simulink model "ModeInputHandle"  (R2018b)
settings: Solver=FixedStepDiscrete  StartTime=0.0  StopTime=10.0  FixedStep=0.01  RelTol=1e-3
undefined symbols (not defined in the file or in its folder): c, CmprtMdHMIReqExt2Tp1, CmprtMdHMIReqExtTp1, CmprtMdHMIReqTp1, d, e, EZESwReq1, f, g, IfVeSMSeStNumConfig, j, KeSMSuButtonLongPressedThrshldTm_Val, KeSMSuFoldType_Val, KeSMSwSeatSMSSeatMdTrigGapTimer_Val, KeSMSwSeatTrigWaitTimer_Val, KeSMSwSRSActiveValidTm_Val, LckUlckActvtFunc1, LstLckFunc1, LugSelectSw1, MdReqTp1, PowerMode1, SeatOccupiedSts1, SRSMode1, StPassCmprtMdCtrl_Md10_VCUConfig_Val, StPassCmprtMdCtrl_Md11_VCUConfig_Val, StPassCmprtMdCtrl_Md12_VCUConfig_Val, StPassCmprtMdCtrl_Md13_VCUConfig_Val, StPassCmprtMdCtrl_Md1_VCUConfig_Val, StPassCmprtMdCtrl_Md27_VCUConfig_Val, StPassCmprtMdCtrl_Md28_VCUConfig_Val, StPassCmprtMdCtrl_Md29_VCUConfig_Val, StPassCmprtMdCtrl_Md2_VCUConfig_Val, StPassCmprtMdCtrl_Md30_VCUConfig_Val, StPassCmprtMdCtrl_Md31_VCUConfig_Val, StPassCmprtMdCtrl_Md32_VCUConfig_Val, StPassCmprtMdCtrl_Md3_VCUConfig_Val, StPassCmprtMdCtrl_Md53_VCUConfig_Val, StPassCmprtMdCtrl_Md56_VCUConfig_Val, StPassCmprtMdCtrl_Md57_VCUConfig_Val, StPassCmprtMdCtrl_Md58_VCUConfig_Val, StPassCmprtMdCtrl_Md61_VCUConfig_Val, StPassCmprtMdCtrl_Md62_VCUConfig_Val, StPassCmprtMdCtrl_Md8_VCUConfig_Val, StPassCmprtMdCtrl_Md9_VCUConfig_Val, StSrv_StMd10_Config_Val, StSrv_StMd11_Config_Val, StSrv_StMd12_Config_Val, StSrv_StMd13_Config_Val, StSrv_StMd1_Config_Val, StSrv_StMd27_Config_Val, StSrv_StMd28_Config_Val, StSrv_StMd29_Config_Val, StSrv_StMd2_Config_Val, StSrv_StMd30_Config_Val, StSrv_StMd31_Config_Val, StSrv_StMd32_Config_Val, StSrv_StMd3_Config_Val, StSrv_StMd8_Config_Val, StSrv_StMd9_Config_Val, VehMovState1
libraries: MSMLib x91
(part 5 of 9)

== system ModeInputHandle/ModelInputHandleRunnable_sys/Subsystem1/AcsEntry4s2RMdReq  ==
  note: // PassAcsEntry4s2RReq ---》 remote
  SwRtRclReq : Inport
  SwRtRclReqV : Inport  Port=2
  AcsEntry4s2RHMI2RRclReq : Inport  Port=3
  PassAcsEntry4s2RReq : Inport  Port=4
  PassCmprtMdHMIReqExt : Inport  Port=5
  SRSSlctSwReq : Inport  Port=6
  SRSCnfmSwReq : Inport  Port=7
  buttonLongPressedThrshhldTm : Inport  Port=8
  curMode : Inport  Port=9
  SRSActiveValidTm : Inport  Port=10
  AcsEntry4s2RAvl : Inport  Port=11
  SRSMode : Inport  Port=12
  AcsEntry4s2RMdConfig : Inport  Port=13
  AND{,1..2,4..5} (5 alike) : Logic  AllPortsSameDT=off  OutDataTypeStr=boolean
  ButtonLongPressed : Subsystem  AncestorBlock=MSMLib/ButtonLongPressed
  ButtonLongPressed2 : Subsystem  AncestorBlock=MSMLib/ButtonLongPressed
  ConfirmRequireSource : MSMLib/ConfirmRequireSource  SystemSampleTime=-1
  Constant : Constant  Value=MdReqTp1.MdReqTp_Start
  Constant1 : Constant  Value=SRSMode1.SRSSlctSwStat_EzeEntry4s2R  OutDataTypeStr=Enum:SRSMode1
  Constant2 : Constant  Value=CmprtMdHMIReqExtTp1.CmprtMdHMIReqExtTp_Mode23  OutDataTypeStr=Enum:CmprtMdHMIReqExtTp1
  Constant3 : Constant  Value=CmprtMdHMIReqExtTp1.CmprtMdHMIReqExtTp_NoAction  OutDataTypeStr=Enum:CmprtMdHMIReqExtTp1
  Constant4 : Constant  Value=true  OutDataTypeStr=boolean
  Constant5 : Constant  Value=0  OutDataTypeStr=uint8
  Constant8 : Constant  Value=9  OutDataTypeStr=uint8
  Equal : RelationalOperator  Operator===  OutDataTypeStr=boolean  RndMeth=Simplest
  Equal1 : RelationalOperator  Operator=~=  OutDataTypeStr=boolean  RndMeth=Simplest
  Equal2 : RelationalOperator  Operator===  OutDataTypeStr=boolean  RndMeth=Simplest
  Equal3 : RelationalOperator  Operator=~=  OutDataTypeStr=boolean  RndMeth=Simplest
  Equal4 : RelationalOperator  Operator===  OutDataTypeStr=boolean  RndMeth=Simplest
  Equal5 : RelationalOperator  Operator=~=  OutDataTypeStr=boolean  RndMeth=Simplest
  Ground2 : Ground
  Logical Operator : Logic  Operator=OR  Inputs=5  AllPortsSameDT=off  OutDataTypeStr=boolean
  NOT : Logic  Operator=NOT  AllPortsSameDT=off  OutDataTypeStr=boolean
  OR1 : Logic  Operator=OR  Inputs=3  AllPortsSameDT=off  OutDataTypeStr=boolean
  Relational Operator3 : RelationalOperator  Operator===  OutDataTypeStr=boolean  RndMeth=Simplest
  SRSReq : MSMLib/SRSReq  SystemSampleTime=-1
  SWIntSrc_S : MSMLib/SWIntSrc_S  SystemSampleTime=-1
  Subsystem4 : MSMLib/MergeReqAndValidity  SystemSampleTime=-1
  Switch1 : Switch  Criteria=u2 > Threshold
  Switch2 : Switch  Criteria=u2 > Threshold
  Unit Delay : UnitDelay  InitialCondition=e  SampleTime=-1
  Unit Delay1 : UnitDelay  InitialCondition=g  SampleTime=-1
  Unit Delay{2..5} (4 alike) : UnitDelay  SampleTime=-1
  Unit Delay6 : UnitDelay  InitialCondition=d  SampleTime=-1
  acsEntry4s2RReq : Outport  VectorParamsAs1DForOutWhenUnconnected=on
  srcReqTp : Outport  Port=2  VectorParamsAs1DForOutWhenUnconnected=on
  SwAcsEntry4s2RIntCnt : Outport  Port=3
  SRSAcsEntry4s2RIntCnt : Outport  Port=4
  Notf1ChimeEventStat : Outport  Port=5
  acsEntry4s2RSoftInt : Outport  Port=6  VectorParamsAs1DForOutWhenUnconnected=on
  wires:
  Unit Delay3/1 -> Equal3/2
  Equal2/1 -> AND5/2
  Constant3/1 -> Equal2/2
  Relational Operator3/1 -> AND5/1
  PassCmprtMdHMIReqExt/1 -> Relational Operator3/1, Unit Delay1/1
  Constant2/1 -> Relational Operator3/2
  Unit Delay1/1 -> Equal2/1
  AND5/1 -> [passCmprtMdHMIReq_AcsEntry4s2R]
  AcsEntry4s2RHMI2RRclReq/1 -> Equal/1, Unit Delay/1
  ButtonLongPressed2/1(mdReq) -> [SRSReq]
  Unit Delay6/1 -> ButtonLongPressed2/6(SRSMode)
  SRSMode/1 -> Unit Delay6/1
  ConfirmRequireSource/1 -> srcReqTp/1
  [HMI2RReq] -> ConfirmRequireSource/3, OR1/1, Logical Operator/2
  OR1/1 -> Switch2/1
  Unit Delay5/1 -> Switch2/3
  Switch2/1 -> acsEntry4s2RSoftInt/1, Unit Delay5/1
  AND4/1 -> Notf1ChimeEventStat/1
  NOT/1 -> AND4/2
  Unit Delay4/1 -> Switch1/3
  Switch1/1 -> acsEntry4s2RReq/1, Unit Delay4/1
  AcsEntry4s2RAvl/1 -> Switch1/2, NOT/1, Switch2/2
  Logical Operator/1 -> Switch1/1, AND4/1
  [PassAcsEntry4s2RReq] -> ConfirmRequireSource/5, OR1/2, Logical Operator/3
  [SRSReq] -> ConfirmRequireSource/6, Logical Operator/5
  [passCmprtMdHMIReq_AcsEntry4s2R] -> ConfirmRequireSource/4, OR1/3, Logical Operator/4
  Unit Delay2/1 -> Equal5/1
  AND2/1 -> [PassAcsEntry4s2RReq]
  Equal5/1 -> AND2/2
  Equal4/1 -> AND2/1
  PassAcsEntry4s2RReq/1 -> Equal4/1, Unit Delay2/1
  Constant4/1 -> Equal5/2, Equal4/2
  AND/1 -> [HMI2RReq]
  [SwMdReq] -> ConfirmRequireSource/1, Logical Operator/1
  Equal1/1 -> AND/2
  Equal/1 -> AND/1
  Unit Delay/1 -> Equal1/1
  Constant/1 -> Equal/2, Equal1/2
  ButtonLongPressed2/2(mdInterruptCnt) -> SRSAcsEntry4s2RIntCnt/1
  SRSReq/1 -> ButtonLongPressed2/1(modeReq)
  SRSActiveValidTm/1 -> SRSReq/2
  Constant1/1 -> ButtonLongPressed2/4(CmpReq), SRSReq/4
  SRSCnfmSwReq/1 -> SRSReq/3, ButtonLongPressed2/5(SRSCnfmSwReq)
  SRSSlctSwReq/1 -> SRSReq/1
  [curMode] -> ButtonLongPressed2/3(curMdState)
  Constant5/1 -> ButtonLongPressed2/2(longPressThrshhldTm)
  curMode/1 -> [curMode]
  buttonLongPressedThrshhldTm/1 -> [buttonLongPressedThrshhldTm]
  ButtonLongPressed/2(mdInterruptCnt) -> SwAcsEntry4s2RIntCnt/1, Unit Delay3/1, Equal3/1
  [buttonLongPressedThrshhldTm] -> ButtonLongPressed/2(longPressThrshhldTm)
  SwRtRclReqV/1 -> Subsystem4/2
  SwRtRclReq/1 -> Subsystem4/1
  ButtonLongPressed/1(mdReq) -> [SwMdReq]
  Ground2/1 -> ConfirmRequireSource/2
  Constant8/1 -> SWIntSrc_S/2
  Equal3/1 -> SWIntSrc_S/1
  AcsEntry4s2RMdConfig/1 -> AND1/1
  Subsystem4/1 -> AND1/2
  AND1/1 -> ButtonLongPressed/1(modeReq)

== system ModeInputHandle/ModelInputHandleRunnable_sys/Subsystem1/AcsEntryAll4sBwdMdReq ==
  AcsEntryAll4sBwdAvl : Inport
  RLDoorAjarSwAct : Inport  Port=2
  RRDoorAjarSwAct : Inport  Port=3
  KeSMSwSeatSMSSeatMdTrigGapTimer : Inport  Port=4
  NotSecRowLeSeaOccStat : Inport  Port=5
  NotSecRowRtSeaOccStat : Inport  Port=6
  Chart : Stateflow chart  TreatAsAtomicUnit=on
  Ground_11 : Ground
  Switch1 : Switch  Criteria=u2 > Threshold
  Switch2 : Switch  Criteria=u2 > Threshold
  Unit Delay4 : UnitDelay  SampleTime=-1
  Unit Delay5 : UnitDelay  SampleTime=-1
  acsEntryAll4sBwdReq : Outport  VectorParamsAs1DForOutWhenUnconnected=on
  acsEntryAll4sBwdSoftInt : Outport  Port=2  VectorParamsAs1DForOutWhenUnconnected=on
  Notf1ChimeEventStat : Outport  Port=3
  acsEntryAll4sBwdReqSig : Outport  Port=4
  wires:
  Ground_11/1 -> Notf1ChimeEventStat/1
  AcsEntryAll4sBwdAvl/1 -> Switch1/2, Switch2/2
  Switch1/1 -> Unit Delay4/1, acsEntryAll4sBwdReq/1
  Unit Delay4/1 -> Switch1/3
  Switch2/1 -> Unit Delay5/1, acsEntryAll4sBwdSoftInt/1
  Unit Delay5/1 -> Switch2/3
  RLDoorAjarSwAct/1 -> Chart/1(iRLDoorAjarSwAct)
  RRDoorAjarSwAct/1 -> Chart/2(iRRDoorAjarSwAct)
  KeSMSwSeatSMSSeatMdTrigGapTimer/1 -> Chart/3(iKeSMSwSeatSMSSeatMdTrigGapTimer)
  NotSecRowLeSeaOccStat/1 -> Chart/4(iNotSecRowLeSeaOccStat)
  NotSecRowRtSeaOccStat/1 -> Chart/5(iNotSecRowRtSeaOccStat)
  Chart/1(oReq) -> acsEntryAll4sBwdReqSig/1, Switch2/1, Switch1/1

== system ModeInputHandle/ModelInputHandleRunnable_sys/Subsystem1/AcsEntryAll4sFwdMdReq ==
  LckUlckActvtFunc : Inport
  NotSecRowLeSeaOccStat : Inport  Port=2
  NotSecRowRtSeaOccStat : Inport  Port=3
  SysPwrMd : Inport  Port=4
  SysPwrMdV : Inport  Port=5
  VehMovState : Inport  Port=6
  AcsEntryAll4sFwdAvl : Inport  Port=7
  LstLckFunc : Inport  Port=8
  LstLckChange : Inport  Port=9
  KeSMSwSeatTrigWaitTimer : Inport  Port=10
  AND : Logic  AllPortsSameDT=off  OutDataTypeStr=boolean
  AND3 : Logic  AllPortsSameDT=off  OutDataTypeStr=boolean
  Chart : Stateflow chart  TreatAsAtomicUnit=on
  Constant : Constant  Value=VehMovState1.VehMvSts_Parked  OutDataTypeStr=Enum: VehMovState1
  Constant1 : Constant  Value=PowerMode1.PowerMode_Off  OutDataTypeStr=Enum: PowerMode1
  Constant10 : Constant  Value=LckUlckActvtFunc1.ActvFunc_VKMdev  OutDataTypeStr=Enum: LckUlckActvtFunc1
  Constant2 : Constant  Value=0  OutDataTypeStr=boolean
  Constant3 : Constant  Value=LstLckFunc1.LstLckFuncTyp_LockAll  OutDataTypeStr=Enum: LstLckFunc1
  Constant4 : Constant  Value=SeatOccupiedSts1.SeatOccupiedSts_Empty  OutDataTypeStr=Enum: SeatOccupiedSts1
  Constant6 : Constant  Value=LckUlckActvtFunc1.ActvFunc_ActvRmtKeyfob  OutDataTypeStr=Enum: LckUlckActvtFunc1
  Constant7 : Constant  Value=LckUlckActvtFunc1.ActvFunc_PasvRmtKeyfob  OutDataTypeStr=Enum: LckUlckActvtFunc1
  Constant8 : Constant  Value=LckUlckActvtFunc1.ActvFunc_EnhancedService  OutDataTypeStr=Enum: LckUlckActvtFunc1
  Constant9 : Constant  Value=LckUlckActvtFunc1.ActvFunc_ExteriorLockSw  OutDataTypeStr=Enum: LckUlckActvtFunc1
  Equal{,1..5,9..13} (11 alike) : RelationalOperator  Operator===  OutDataTypeStr=boolean  RndMeth=Simplest
  Equal6 : RelationalOperator  Operator=~=  OutDataTypeStr=boolean  RndMeth=Simplest
  Ground_11 : Ground
  OR3 : Logic  Operator=OR  Inputs=5  AllPortsSameDT=off  OutDataTypeStr=boolean
  Switch1 : Switch  Criteria=u2 > Threshold
  Switch2 : Switch  Criteria=u2 > Threshold
  Unit Delay : UnitDelay  SampleTime=-1
  Unit Delay4 : UnitDelay  SampleTime=-1
  Unit Delay5 : UnitDelay  SampleTime=-1
  acsEntryAll4sFwdReq : Outport  VectorParamsAs1DForOutWhenUnconnected=on
  acsEntryAll4sFwdSoftInt : Outport  Port=2  VectorParamsAs1DForOutWhenUnconnected=on
  Notf1ChimeEventStat : Outport  Port=3
  "acsEntryAll4sFwdReqSig " : Outport  Port=4
  wires:
  Unit Delay5/1 -> Switch2/3
  Switch2/1 -> acsEntryAll4sFwdSoftInt/1, Unit Delay5/1
  Unit Delay4/1 -> Switch1/3
  Switch1/1 -> acsEntryAll4sFwdReq/1, Unit Delay4/1
  AcsEntryAll4sFwdAvl/1 -> Switch2/2, Switch1/2
  VehMovState/1 -> Equal/1
  Constant/1 -> Equal/2
  SysPwrMd/1 -> Equal1/1
  Constant1/1 -> Equal1/2
  Constant2/1 -> Equal2/2
  SysPwrMdV/1 -> Equal2/1
  NotSecRowLeSeaOccStat/1 -> Equal3/1
  LckUlckActvtFunc/1 -> Equal13/1, Equal12/1, Equal11/1, Equal10/1, Equal9/1
  Constant6/1 -> Equal9/2
  Constant7/1 -> Equal10/2
  Constant8/1 -> Equal11/2
  Constant9/1 -> Equal12/2
  Constant10/1 -> Equal13/2
  Equal9/1 -> OR3/1
  Equal10/1 -> OR3/2
  Equal11/1 -> OR3/3
  Equal12/1 -> OR3/4
  Equal13/1 -> OR3/5
  Equal1/1 -> AND3/1
  Equal2/1 -> AND3/2
  Ground_11/1 -> Notf1ChimeEventStat/1
  Constant4/1 -> Equal4/1, Equal3/2
  NotSecRowRtSeaOccStat/1 -> Equal4/2
  Equal3/1 -> AND/1
  Equal4/1 -> AND/2
  LstLckFunc/1 -> Equal5/1
  Constant3/1 -> Equal5/2
  LstLckChange/1 -> Unit Delay/1, Equal6/1
  Unit Delay/1 -> Equal6/2
  Chart/1(AcsEntryAll4sFwdMdV) -> "acsEntryAll4sFwdReqSig "/1, Switch2/1, Switch1/1
  Equal/1 -> Chart/1(ibVehMovState)
  AND3/1 -> Chart/2(ibSysPwrMd)
  Equal5/1 -> Chart/3(ibLstLckFunc)
  Equal6/1 -> Chart/4(ibLstLckChange)
  OR3/1 -> Chart/5(ibLckUlckActvtFunc)
  AND/1 -> Chart/6(ibNotSecRowLRSeaOccEmpty)
  KeSMSwSeatTrigWaitTimer/1 -> Chart/7(iKeSMSwSeatTrigWaitTimer)

== system ModeInputHandle/ModelInputHandleRunnable_sys/Subsystem1/AcsEntryMdReq ==
  note: // PassAcsMdEtryReq---》 remote
  AcsMdExtSwLtRclReq : Inport
  AcsMdExtSwLtRclReqV : Inport  Port=2
  AcsMdExtSwRtRclReq : Inport  Port=3
  AcsMdExtSwRtRclReqV : Inport  Port=4
  PassAcsMdEtryReq : Inport  Port=5
  passCmprtMdHMIReq : Inport  Port=6
  SRSSlctSwReq : Inport  Port=7
  SRSCnfmSwReq : Inport  Port=8
  buttonLongPressedThrshhldTm : Inport  Port=9
  curMode : Inport  Port=10
  SRSActiveValidTm : Inport  Port=11
  AcsMdEntyAvl : Inport  Port=12
  SRSMode : Inport  Port=13
  RrRcvyMdSwRclReq : Inport  Port=14
  RrRcvyMdSwRclReqV : Inport  Port=15
  HMI2LRclReq : Inport  Port=16
  HMI2RRclReq : Inport  Port=17
  StPassCmprtMdCtrl_Md1_VCUConfig : Inport  Port=18
  StSrv_StMd1_Config : Inport  Port=19
  AND : Logic  AllPortsSameDT=off  OutDataTypeStr=boolean
  AND1 : Logic  Commented=on  AllPortsSameDT=off  OutDataTypeStr=boolean
  AND2 : Logic  AllPortsSameDT=off  OutDataTypeStr=boolean
  AND3 : Logic  AllPortsSameDT=off  OutDataTypeStr=boolean
  AND4 : Logic  Commented=on  AllPortsSameDT=off  OutDataTypeStr=boolean
  ButtonLongPressed1 : Subsystem  AncestorBlock=MSMLib/ButtonLongPressed
  ButtonLongPressed2 : Subsystem  Commented=on  AncestorBlock=MSMLib/ButtonLongPressed
  ButtonLongPressed3 : Subsystem  AncestorBlock=MSMLib/ButtonLongPressed
  ButtonLongPressed4 : Subsystem  AncestorBlock=MSMLib/ButtonLongPressed
  ConfirmRequireSource : MSMLib/ConfirmRequireSource  SystemSampleTime=-1
  Constant : Constant  Commented=on  Value=MdReqTp1.MdReqTp_Start
  Constant1 : Constant  Commented=on  Value=SRSMode1.SRSSlctSwStat_EzeEntry  OutDataTypeStr=Enum:SRSMode1
  Constant13 : Constant  OutDataTypeStr=uint8
  Constant2 : Constant  Value=CmprtMdHMIReqTp1.CmprtMdHMIReqTp_Mode1  OutDataTypeStr=Enum:CmprtMdHMIReqTp1
  Constant3 : Constant  Value=0  OutDataTypeStr=boolean
  Constant4 : Constant  Value=true  OutDataTypeStr=boolean
  Constant5 : Constant  Commented=on  Value=0  OutDataTypeStr=uint8
  Constant6 : Constant  Value=0  OutDataTypeStr=boolean
  Constant7 : Constant  Commented=on  Value=MdReqTp1.MdReqTp_Start
  Constant8 : Constant  Value=CmprtMdHMIReqTp1.CmprtMdHMIReqTp_NoAction  OutDataTypeStr=Enum:CmprtMdHMIReqTp1
  Equal : RelationalOperator  Commented=on  Operator===  OutDataTypeStr=boolean  RndMeth=Simplest
  Equal1 : RelationalOperator  Commented=on  Operator=~=  OutDataTypeStr=boolean  RndMeth=Simplest
  Equal{5,8..11} (5 alike) : RelationalOperator  Operator=~=  OutDataTypeStr=boolean  RndMeth=Simplest
  Equal2 : RelationalOperator  Commented=on  Operator===  OutDataTypeStr=boolean  RndMeth=Simplest
  Equal3 : RelationalOperator  Commented=on  Operator=~=  OutDataTypeStr=boolean  RndMeth=Simplest
  Equal4 : RelationalOperator  Operator===  OutDataTypeStr=boolean  RndMeth=Simplest
  Equal6 : RelationalOperator  Operator===  OutDataTypeStr=boolean  RndMeth=Simplest
  From5 : From  Commented=on  GotoTag=curMode
  Goto10 : Goto  Commented=on  GotoTag=SRSReq
  Goto6 : Goto  Commented=on  GotoTag=HMI2RReq
  Goto7 : Goto  Commented=on  GotoTag=HMI2LReq
  Ground1 : Ground
  Ground84 : Ground
  Logical Operator : Logic  Operator=OR  Inputs=3  AllPortsSameDT=off  OutDataTypeStr=boolean
  Logical Operator1 : Logic  Operator=OR  Inputs=3  AllPortsSameDT=off  OutDataTypeStr=boolean
  NOT : Logic  Operator=NOT  AllPortsSameDT=off  OutDataTypeStr=boolean
  OR : Logic  Operator=OR  Inputs=3  AllPortsSameDT=off  OutDataTypeStr=boolean
  OR1 : Logic  Operator=OR  AllPortsSameDT=off  OutDataTypeStr=boolean
  Relational Operator : RelationalOperator  Operator===  OutDataTypeStr=boolean  RndMeth=Simplest
  SRSReq : MSMLib/SRSReq  Commented=on  SystemSampleTime=-1
  SWIntSrc : MSMLib/SWIntSrc  SystemSampleTime=-1
  Subsystem1 : MSMLib/MergeReqAndValidity  SystemSampleTime=-1
  Subsystem2 : MSMLib/MergeReqAndValidity  SystemSampleTime=-1
  Subsystem3 : MSMLib/MergeReqAndValidity  SystemSampleTime=-1
  Switch{,1..3} (4 alike) : Switch  Criteria=u2 > Threshold
  Terminator_{1..5,69} (6 alike) : Terminator
  Unit Delay{,1..2,8..11} (7 alike) : UnitDelay  SampleTime=-1
  Unit Delay3 : UnitDelay  InitialCondition=c  SampleTime=-1
  Unit Delay4 : UnitDelay  Commented=on  InitialCondition=d  SampleTime=-1
  Unit Delay5 : UnitDelay  Commented=on  InitialCondition=e  SampleTime=-1
  Unit Delay6 : UnitDelay  Commented=on  InitialCondition=e  SampleTime=-1
  acsEntyMdReq : Outport  VectorParamsAs1DForOutWhenUnconnected=on
  srcReqTp : Outport  Port=2  VectorParamsAs1DForOutWhenUnconnected=on
  "SwAcsEntyLIntCnt " : Outport  Port=3
  acsEntySoftInt : Outport  Port=4
  SRSAcsEntyIntCnt : Outport  Port=5
  Notf1ChimeEventStat : Outport  Port=6
  SwAcsEntyRIntCnt : Outport  Port=7
  SwAcsEntyBIntCnt : Outport  Port=8
  wires:
  curMode/1 -> [curMode]
  [buttonLongPressedThrshhldTm] -> ButtonLongPressed1/2(longPressThrshhldTm)
  ButtonLongPressed1/2(mdInterruptCnt) -> "SwAcsEntyLIntCnt "/1, Unit Delay8/1, Equal8/1
  Logical Operator1/1 -> [SwMdReq]
  Equal5/1 -> AND2/2
  Unit Delay3/1 -> Equal6/1
  Equal6/1 -> AND3/2
  PassAcsMdEtryReq/1 -> Unit Delay2/1, Equal4/1
  Constant4/1 -> Equal4/2, Equal5/2
  Relational Operator/1 -> AND3/1
  Equal4/1 -> AND2/1
  Unit Delay2/1 -> Equal5/1
  Constant1/1 -> ButtonLongPressed2/4(CmpReq), SRSReq/4
  Constant5/1 -> ButtonLongPressed2/2(longPressThrshhldTm)
  SRSReq/1 -> ButtonLongPressed2/1(modeReq)
  From5/1 -> ButtonLongPressed2/3(curMdState)
  buttonLongPressedThrshhldTm/1 -> [buttonLongPressedThrshhldTm]
  [SwMdReq] -> Logical Operator/1, ConfirmRequireSource/1
  [PassAcsMdEtryReq] -> OR1/1, Logical Operator/2, ConfirmRequireSource/5
  [passCmprtMdHMIReq] -> Logical Operator/3, OR1/2, ConfirmRequireSource/4
  AcsMdEntyAvl/1 -> Switch2/2, NOT/1, Switch1/2
  Logical Operator/1 -> AND/1, Switch1/1
  Switch1/1 -> Unit Delay/1, acsEntyMdReq/1
  Unit Delay/1 -> Switch1/3
  NOT/1 -> AND/2
  AND/1 -> Notf1ChimeEventStat/1
  OR1/1 -> Switch2/1
  Switch2/1 -> acsEntySoftInt/1, Unit Delay1/1
  Unit Delay1/1 -> Switch2/3
  ButtonLongPressed2/1(mdReq) -> Goto10/1
  Unit Delay4/1 -> ButtonLongPressed2/6(SRSMode)
  passCmprtMdHMIReq/1 -> Unit Delay3/1, Relational Operator/1
  Constant2/1 -> Relational Operator/2
  [buttonLongPressedThrshhldTm] -> ButtonLongPressed3/2(longPressThrshhldTm)
  ButtonLongPressed3/2(mdInterruptCnt) -> SwAcsEntyBIntCnt/1, Unit Delay9/1, Equal9/1
  RrRcvyMdSwRclReq/1 -> Subsystem1/1
  RrRcvyMdSwRclReqV/1 -> Subsystem1/2
  Subsystem1/1 -> ButtonLongPressed3/1(modeReq)
  ConfirmRequireSource/1 -> srcReqTp/1
  Equal3/1 -> AND4/2
  AND4/1 -> Goto6/1
  Unit Delay5/1 -> Equal1/1
  Constant/1 -> Equal1/2, Equal/2
  Constant7/1 -> Equal3/2, Equal2/2
  Unit Delay6/1 -> Equal3/1
  Equal1/1 -> AND1/2
  Equal2/1 -> AND4/1
  Equal/1 -> AND1/1
  AND1/1 -> Goto7/1
  Subsystem2/1 -> ButtonLongPressed1/1(modeReq)
  AcsMdExtSwLtRclReq/1 -> Subsystem2/1
  AcsMdExtSwLtRclReqV/1 -> Subsystem2/2
  Constant8/1 -> Equal6/2
  Unit Delay8/1 -> Equal8/2
  Unit Delay9/1 -> Equal9/2
  OR/1 -> Unit Delay10/1, Equal10/1, SWIntSrc/1
  Unit Delay10/1 -> Equal10/2
  Equal10/1 -> SWIntSrc/2
  Constant13/1 -> SWIntSrc/3
  Subsystem3/1 -> ButtonLongPressed4/1(modeReq)
  AcsMdExtSwRtRclReqV/1 -> Subsystem3/2
  AcsMdExtSwRtRclReq/1 -> Subsystem3/1
  [buttonLongPressedThrshhldTm] -> ButtonLongPressed4/2(longPressThrshhldTm)
  Unit Delay11/1 -> Equal11/2
  ButtonLongPressed4/2(mdInterruptCnt) -> Equal11/1, Unit Delay11/1, SwAcsEntyRIntCnt/1
  ButtonLongPressed4/1(mdReq) -> Logical Operator1/1
  ButtonLongPressed1/1(mdReq) -> Logical Operator1/2
  ButtonLongPressed3/1(mdReq) -> Logical Operator1/3
  Equal11/1 -> OR/1
  Equal8/1 -> OR/2
  Equal9/1 -> OR/3
  HMI2LRclReq/1 -> Terminator_69/1
  HMI2RRclReq/1 -> Terminator_1/1
  SRSSlctSwReq/1 -> Terminator_2/1
  SRSActiveValidTm/1 -> Terminator_3/1
  SRSCnfmSwReq/1 -> Terminator_4/1
  SRSMode/1 -> Terminator_5/1
  Ground84/1 -> SRSAcsEntyIntCnt/1
  Ground1/1 -> ConfirmRequireSource/6, ConfirmRequireSource/3, ConfirmRequireSource/2
  AND2/1 -> Switch/1
  Switch/1 -> [PassAcsMdEtryReq]
  StSrv_StMd1_Config/1 -> Switch/2
  Constant3/1 -> Switch/3
  StPassCmprtMdCtrl_Md1_VCUConfig/1 -> Switch3/2
  AND3/1 -> Switch3/1
  Switch3/1 -> [passCmprtMdHMIReq]
  Constant6/1 -> Switch3/3

== system ModeInputHandle/ModelInputHandleRunnable_sys/Subsystem1/AcsExit4s2LMdReq ==
  note: // PassAcsExit4s2LReq ---》 remote
  EZE4SSwReq : Inport
  AcsExit4s2LHMI2LRclReq : Inport  Port=2
  PassAcsExit4s2LReq : Inport  Port=3
  PassCmprtMdHMIReqExt : Inport  Port=4
  SRSSlctSwReq : Inport  Port=5
  SRSCnfmSwReq : Inport  Port=6
  buttonLongPressedThrshhldTm : Inport  Port=7
  curMode : Inport  Port=8
  SRSActiveValidTm : Inport  Port=9
  AcsExit4s2LAvl : Inport  Port=10
  SRSMode : Inport  Port=11
  AND{,2,4..5} (4 alike) : Logic  AllPortsSameDT=off  OutDataTypeStr=boolean
  ButtonLongPressed2 : Subsystem  AncestorBlock=MSMLib/ButtonLongPressed
  ButtonLongPressed3 : Subsystem  AncestorBlock=MSMLib/ButtonLongPressed
  ConfirmRequireSource : MSMLib/ConfirmRequireSource  SystemSampleTime=-1
  Constant : Constant  Value=MdReqTp1.MdReqTp_Start
  Constant1 : Constant  Value=SRSMode1.SRSSlctSwStat_EzeExt4s2L  OutDataTypeStr=Enum:SRSMode1
  Constant2 : Constant  Value=CmprtMdHMIReqExtTp1.CmprtMdHMIReqExtTp_Mode22  OutDataTypeStr=Enum:CmprtMdHMIReqExtTp1
  Constant3 : Constant  Value=CmprtMdHMIReqExtTp1.CmprtMdHMIReqExtTp_NoAction  OutDataTypeStr=Enum:CmprtMdHMIReqExtTp1
  Constant4 : Constant  Value=true  OutDataTypeStr=boolean
  Constant5 : Constant  Value=0  OutDataTypeStr=uint8
  Constant8 : Constant  Value=8  OutDataTypeStr=uint8
  Constant9 : Constant  Value=EZESwReq1.EZE_OUT  OutDataTypeStr=Enum: EZESwReq1
  Equal{,2,4,6} (4 alike) : RelationalOperator  Operator===  OutDataTypeStr=boolean  RndMeth=Simplest
  Equal1 : RelationalOperator  Operator=~=  OutDataTypeStr=boolean  RndMeth=Simplest
  Equal3 : RelationalOperator  Operator=~=  OutDataTypeStr=boolean  RndMeth=Simplest
  Equal5 : RelationalOperator  Operator=~=  OutDataTypeStr=boolean  RndMeth=Simplest
  Ground2 : Ground
  Logical Operator : Logic  Operator=OR  Inputs=5  AllPortsSameDT=off  OutDataTypeStr=boolean
  NOT : Logic  Operator=NOT  AllPortsSameDT=off  OutDataTypeStr=boolean
  OR1 : Logic  Operator=OR  Inputs=3  AllPortsSameDT=off  OutDataTypeStr=boolean
  Relational Operator3 : RelationalOperator  Operator===  OutDataTypeStr=boolean  RndMeth=Simplest
  SRSReq : MSMLib/SRSReq  SystemSampleTime=-1
  SWIntSrc_S : MSMLib/SWIntSrc_S  SystemSampleTime=-1
  Switch1 : Switch  Criteria=u2 > Threshold
  Switch2 : Switch  Criteria=u2 > Threshold
  Unit Delay : UnitDelay  InitialCondition=e  SampleTime=-1
  Unit Delay1 : UnitDelay  InitialCondition=g  SampleTime=-1
  Unit Delay{2..5} (4 alike) : UnitDelay  SampleTime=-1
  Unit Delay6 : UnitDelay  InitialCondition=d  SampleTime=-1
  acsExit4s2LReq : Outport  VectorParamsAs1DForOutWhenUnconnected=on
  srcReqTp : Outport  Port=2  VectorParamsAs1DForOutWhenUnconnected=on
  "SwAcsExit4s2LIntCnt " : Outport  Port=3
  SRSAcsExit4s2LIntCnt : Outport  Port=4
  Notf1ChimeEventStat : Outport  Port=5
  acsExit4s2LSoftInt : Outport  Port=6  VectorParamsAs1DForOutWhenUnconnected=on
  wires:
  Equal6/1 -> ButtonLongPressed3/1(modeReq)
  Constant9/1 -> Equal6/2
  EZE4SSwReq/1 -> Equal6/1
  Ground2/1 -> ConfirmRequireSource/3
  ButtonLongPressed3/2(mdInterruptCnt) -> "SwAcsExit4s2LIntCnt "/1, Unit Delay3/1, Equal3/1
  Equal3/1 -> SWIntSrc_S/1
  Unit Delay3/1 -> Equal3/2
  ButtonLongPressed3/1(mdReq) -> [SwMdReq]
  [buttonLongPressedThrshhldTm] -> ButtonLongPressed3/2(longPressThrshhldTm)
  Equal2/1 -> AND5/2
  Constant3/1 -> Equal2/2
  Relational Operator3/1 -> AND5/1
  PassCmprtMdHMIReqExt/1 -> Relational Operator3/1, Unit Delay1/1
  Constant2/1 -> Relational Operator3/2
  Unit Delay1/1 -> Equal2/1
  AND5/1 -> [passCmprtMdHMIReq_AcsExit4s2L]
  AcsExit4s2LHMI2LRclReq/1 -> Equal/1, Unit Delay/1
  ButtonLongPressed2/1(mdReq) -> [SRSReq]
  Unit Delay6/1 -> ButtonLongPressed2/6(SRSMode)
  SRSMode/1 -> Unit Delay6/1
  ConfirmRequireSource/1 -> srcReqTp/1
  [HMI2LReq] -> OR1/1, ConfirmRequireSource/2, Logical Operator/2
  OR1/1 -> Switch2/1
  Unit Delay5/1 -> Switch2/3
  Switch2/1 -> acsExit4s2LSoftInt/1, Unit Delay5/1
  AND4/1 -> Notf1ChimeEventStat/1
  NOT/1 -> AND4/2
  Unit Delay4/1 -> Switch1/3
  Switch1/1 -> acsExit4s2LReq/1, Unit Delay4/1
  AcsExit4s2LAvl/1 -> Switch1/2, NOT/1, Switch2/2
  Logical Operator/1 -> Switch1/1, AND4/1
  [PassAcsExit4s2LReq] -> ConfirmRequireSource/5, OR1/2, Logical Operator/3
  [SRSReq] -> ConfirmRequireSource/6, Logical Operator/5
  [passCmprtMdHMIReq_AcsExit4s2L] -> ConfirmRequireSource/4, OR1/3, Logical Operator/4
  Unit Delay2/1 -> Equal5/1
  AND2/1 -> [PassAcsExit4s2LReq]
  Equal5/1 -> AND2/2
  Equal4/1 -> AND2/1
  PassAcsExit4s2LReq/1 -> Equal4/1, Unit Delay2/1
  Constant4/1 -> Equal5/2, Equal4/2
  AND/1 -> [HMI2LReq]
  [SwMdReq] -> ConfirmRequireSource/1, Logical Operator/1
  Equal1/1 -> AND/2
  Equal/1 -> AND/1
  Unit Delay/1 -> Equal1/1
  Constant/1 -> Equal/2, Equal1/2
  ButtonLongPressed2/2(mdInterruptCnt) -> SRSAcsExit4s2LIntCnt/1
  SRSReq/1 -> ButtonLongPressed2/1(modeReq)
  SRSActiveValidTm/1 -> SRSReq/2
  Constant1/1 -> ButtonLongPressed2/4(CmpReq), SRSReq/4
  SRSCnfmSwReq/1 -> SRSReq/3, ButtonLongPressed2/5(SRSCnfmSwReq)
  SRSSlctSwReq/1 -> SRSReq/1
  [curMode] -> ButtonLongPressed2/3(curMdState)
  Constant5/1 -> ButtonLongPressed2/2(longPressThrshhldTm)
  curMode/1 -> [curMode]
  buttonLongPressedThrshhldTm/1 -> [buttonLongPressedThrshhldTm]
  Constant8/1 -> SWIntSrc_S/2

== system ModeInputHandle/ModelInputHandleRunnable_sys/Subsystem1/AcsExit4s2RMdReq ==
  note: // PassAcsExit4s2RReq ---》 remote
  AcsMdExt4SSwRtRclReq : Inport
  AcsMdExt4SSwRtRclReqV : Inport  Port=2
  AcsExit4s2RHMI2RRclReq : Inport  Port=3
  PassAcsExit4s2RReq : Inport  Port=4
  PassCmprtMdHMIReqExt : Inport  Port=5
  SRSSlctSwReq : Inport  Port=6
  SRSCnfmSwReq : Inport  Port=7
  buttonLongPressedThrshhldTm : Inport  Port=8
  curMode : Inport  Port=9
  SRSActiveValidTm : Inport  Port=10
  AcsExit4s2RAvl : Inport  Port=11
  SRSMode : Inport  Port=12
  AND{,2,4..5} (4 alike) : Logic  AllPortsSameDT=off  OutDataTypeStr=boolean
  ButtonLongPressed : Subsystem  AncestorBlock=MSMLib/ButtonLongPressed
  ButtonLongPressed2 : Subsystem  AncestorBlock=MSMLib/ButtonLongPressed
  ConfirmRequireSource : MSMLib/ConfirmRequireSource  SystemSampleTime=-1
  Constant : Constant  Value=MdReqTp1.MdReqTp_Start
  Constant1 : Constant  Value=SRSMode1.SRSSlctSwStat_EzeExt4s2R  OutDataTypeStr=Enum:SRSMode1
  Constant2 : Constant  Value=CmprtMdHMIReqExtTp1.CmprtMdHMIReqExtTp_Mode24  OutDataTypeStr=Enum:CmprtMdHMIReqExtTp1
  Constant3 : Constant  Value=CmprtMdHMIReqExtTp1.CmprtMdHMIReqExtTp_NoAction  OutDataTypeStr=Enum:CmprtMdHMIReqExtTp1
  Constant4 : Constant  Value=true  OutDataTypeStr=boolean
  Constant5 : Constant  Value=0  OutDataTypeStr=uint8
  Constant8 : Constant  Value=10  OutDataTypeStr=uint8
  Equal : RelationalOperator  Operator===  OutDataTypeStr=boolean  RndMeth=Simplest
  Equal1 : RelationalOperator  Operator=~=  OutDataTypeStr=boolean  RndMeth=Simplest
  Equal2 : RelationalOperator  Operator===  OutDataTypeStr=boolean  RndMeth=Simplest
  Equal3 : RelationalOperator  Operator=~=  OutDataTypeStr=boolean  RndMeth=Simplest
  Equal4 : RelationalOperator  Operator===  OutDataTypeStr=boolean  RndMeth=Simplest
  Equal5 : RelationalOperator  Operator=~=  OutDataTypeStr=boolean  RndMeth=Simplest
  Ground2 : Ground
  Logical Operator : Logic  Operator=OR  Inputs=5  AllPortsSameDT=off  OutDataTypeStr=boolean
  NOT : Logic  Operator=NOT  AllPortsSameDT=off  OutDataTypeStr=boolean
  OR1 : Logic  Operator=OR  Inputs=3  AllPortsSameDT=off  OutDataTypeStr=boolean
  Relational Operator3 : RelationalOperator  Operator===  OutDataTypeStr=boolean  RndMeth=Simplest
  SRSReq : MSMLib/SRSReq  SystemSampleTime=-1
  SWIntSrc_S : MSMLib/SWIntSrc_S  SystemSampleTime=-1
  Subsystem4 : MSMLib/MergeReqAndValidity  SystemSampleTime=-1
  Switch1 : Switch  Criteria=u2 > Threshold
  Switch2 : Switch  Criteria=u2 > Threshold
  Unit Delay : UnitDelay  InitialCondition=e  SampleTime=-1
  Unit Delay1 : UnitDelay  InitialCondition=g  SampleTime=-1
  Unit Delay{2..5} (4 alike) : UnitDelay  SampleTime=-1
  Unit Delay6 : UnitDelay  InitialCondition=d  SampleTime=-1
  acsExit4s2RReq : Outport  VectorParamsAs1DForOutWhenUnconnected=on
  srcReqTp : Outport  Port=2  VectorParamsAs1DForOutWhenUnconnected=on
  SwAcsExit4s2RIntCnt : Outport  Port=3
  SRSAcsExit4s2RIntCnt : Outport  Port=4
  Notf1ChimeEventStat : Outport  Port=5
  acsExit4s2RSoftInt : Outport  Port=6  VectorParamsAs1DForOutWhenUnconnected=on
  wires:
  Ground2/1 -> ConfirmRequireSource/2
  ButtonLongPressed/1(mdReq) -> [SwMdReq]
  AcsMdExt4SSwRtRclReq/1 -> Subsystem4/1
  AcsMdExt4SSwRtRclReqV/1 -> Subsystem4/2
  Subsystem4/1 -> ButtonLongPressed/1(modeReq)
  [buttonLongPressedThrshhldTm] -> ButtonLongPressed/2(longPressThrshhldTm)
  ButtonLongPressed/2(mdInterruptCnt) -> Equal3/1, Unit Delay3/1, SwAcsExit4s2RIntCnt/1
  buttonLongPressedThrshhldTm/1 -> [buttonLongPressedThrshhldTm]
  curMode/1 -> [curMode]
  Constant5/1 -> ButtonLongPressed2/2(longPressThrshhldTm)
  [curMode] -> ButtonLongPressed2/3(curMdState)
  SRSSlctSwReq/1 -> SRSReq/1
  SRSCnfmSwReq/1 -> ButtonLongPressed2/5(SRSCnfmSwReq), SRSReq/3
  Constant1/1 -> SRSReq/4, ButtonLongPressed2/4(CmpReq)
  SRSActiveValidTm/1 -> SRSReq/2
  SRSReq/1 -> ButtonLongPressed2/1(modeReq)
  ButtonLongPressed2/2(mdInterruptCnt) -> SRSAcsExit4s2RIntCnt/1
  Constant/1 -> Equal1/2, Equal/2
  Unit Delay/1 -> Equal1/1
  Equal/1 -> AND/1
  Equal1/1 -> AND/2
  [SwMdReq] -> Logical Operator/1, ConfirmRequireSource/1
  AND/1 -> [HMI2RReq]
  Constant4/1 -> Equal4/2, Equal5/2
  PassAcsExit4s2RReq/1 -> Unit Delay2/1, Equal4/1
  Equal4/1 -> AND2/1
  Equal5/1 -> AND2/2
  AND2/1 -> [PassAcsExit4s2RReq]
  Unit Delay2/1 -> Equal5/1
  [passCmprtMdHMIReq_AcsExit4s2R] -> Logical Operator/4, OR1/3, ConfirmRequireSource/4
  [SRSReq] -> Logical Operator/5, ConfirmRequireSource/6
  [PassAcsExit4s2RReq] -> Logical Operator/3, OR1/2, ConfirmRequireSource/5
  Logical Operator/1 -> AND4/1, Switch1/1
  AcsExit4s2RAvl/1 -> Switch2/2, NOT/1, Switch1/2
  Switch1/1 -> Unit Delay4/1, acsExit4s2RReq/1
  Unit Delay4/1 -> Switch1/3
  NOT/1 -> AND4/2
  AND4/1 -> Notf1ChimeEventStat/1
  Switch2/1 -> Unit Delay5/1, acsExit4s2RSoftInt/1
  Unit Delay5/1 -> Switch2/3
  OR1/1 -> Switch2/1
  [HMI2RReq] -> Logical Operator/2, OR1/1, ConfirmRequireSource/3
  ConfirmRequireSource/1 -> srcReqTp/1
  SRSMode/1 -> Unit Delay6/1
  Unit Delay6/1 -> ButtonLongPressed2/6(SRSMode)
  ButtonLongPressed2/1(mdReq) -> [SRSReq]
  AcsExit4s2RHMI2RRclReq/1 -> Unit Delay/1, Equal/1
  AND5/1 -> [passCmprtMdHMIReq_AcsExit4s2R]
  Unit Delay1/1 -> Equal2/1
  Constant2/1 -> Relational Operator3/2
  PassCmprtMdHMIReqExt/1 -> Unit Delay1/1, Relational Operator3/1
  Relational Operator3/1 -> AND5/1
  Constant3/1 -> Equal2/2
  Equal2/1 -> AND5/2
  Unit Delay3/1 -> Equal3/2
  Equal3/1 -> SWIntSrc_S/1
  Constant8/1 -> SWIntSrc_S/2

== system ModeInputHandle/ModelInputHandleRunnable_sys/Subsystem1/AcsExtMdReq ==
  note: // PassAcsMdExt ---》 remote
  SwRtRclReq : Inport  OutDataTypeStr=boolean
  SwRtRclReqV : Inport  Port=2
  SwLtRclReq : Inport  Port=3  OutDataTypeStr=boolean
  SwLtRclReqV : Inport  Port=4
  HMI2LRclReq : Inport  Port=5
  HMI2RRclReq : Inport  Port=6
  PassAcsMdExtReq : Inport  Port=7
  passCmprtMdHMIReq : Inport  Port=8
  SRSSlctSwReq : Inport  Port=9
  SRSCnfmSwReq : Inport  Port=10
  buttonLongPressedThrshhldTm : Inport  Port=11
  curMode : Inport  Port=12
  SRSActiveValidTm : Inport  Port=13
  AcsMdExtAvl : Inport  Port=14
  SRSMode : Inport  Port=15
  AND{,1..4} (5 alike) : Logic  AllPortsSameDT=off  OutDataTypeStr=boolean
  ButtonLongPressed : Subsystem  AncestorBlock=MSMLib/ButtonLongPressed
  ButtonLongPressed1 : Subsystem  AncestorBlock=MSMLib/ButtonLongPressed
  ButtonLongPressed2 : Subsystem  AncestorBlock=MSMLib/ButtonLongPressed
  ConfirmRequireSource : MSMLib/ConfirmRequireSource  SystemSampleTime=-1
  Constant : Constant  Value=MdReqTp1.MdReqTp_Start
  Constant1 : Constant  Value=SRSMode1.SRSSlctSwStat_EzeExt  OutDataTypeStr=Enum:SRSMode1
  Constant11 : Constant  Value=0  OutDataTypeStr=uint8
  Constant2 : Constant  Value=CmprtMdHMIReqTp1.CmprtMdHMIReqTp_Mode4  OutDataTypeStr=Enum:CmprtMdHMIReqTp1
  Constant3 : Constant  Value=MdReqTp1.MdReqTp_Start
  Constant4 : Constant  Value=true  OutDataTypeStr=boolean
  Constant5 : Constant  Value=0  OutDataTypeStr=uint8
  Constant8 : Constant  Value=CmprtMdHMIReqTp1.CmprtMdHMIReqTp_NoAction  OutDataTypeStr=Enum:CmprtMdHMIReqTp1
  Equal{,2,4,6} (4 alike) : RelationalOperator  Operator===  OutDataTypeStr=boolean  RndMeth=Simplest
  Equal{1,3,5,7..9} (6 alike) : RelationalOperator  Operator=~=  OutDataTypeStr=boolean  RndMeth=Simplest
  Logical Operator : Logic  Operator=OR  Inputs=6  AllPortsSameDT=off  OutDataTypeStr=boolean
  Logical Operator1 : Logic  Operator=OR  AllPortsSameDT=off  OutDataTypeStr=boolean
  NOT : Logic  Operator=NOT  AllPortsSameDT=off  OutDataTypeStr=boolean
  OR : Logic  Operator=OR  AllPortsSameDT=off  OutDataTypeStr=boolean
  OR1 : Logic  Operator=OR  Inputs=4  AllPortsSameDT=off  OutDataTypeStr=boolean
  Relational Operator : RelationalOperator  Operator===  OutDataTypeStr=boolean  RndMeth=Simplest
  SRSReq : MSMLib/SRSReq  SystemSampleTime=-1
  SWIntSrc : MSMLib/SWIntSrc  SystemSampleTime=-1
  Subsystem1 : MSMLib/MergeReqAndValidity  SystemSampleTime=-1
  Subsystem4 : MSMLib/MergeReqAndValidity  SystemSampleTime=-1
  Switch1 : Switch  Criteria=u2 > Threshold
  Switch2 : Switch  Criteria=u2 > Threshold
  Unit Delay : UnitDelay  InitialCondition=e  SampleTime=-1
  Unit Delay1 : UnitDelay  InitialCondition=e  SampleTime=-1
  Unit Delay{2,4..5,7..9} (6 alike) : UnitDelay  SampleTime=-1
  Unit Delay3 : UnitDelay  InitialCondition=c  SampleTime=-1
  Unit Delay6 : UnitDelay  InitialCondition=d  SampleTime=-1
  acsExtMdReq : Outport  VectorParamsAs1DForOutWhenUnconnected=on
  srcReqTp : Outport  Port=2  VectorParamsAs1DForOutWhenUnconnected=on
  "SwAcsExtLIntCnt " : Outport  Port=3
  SRSRclIntCnt : Outport  Port=4
  Notf1ChimeEventStat : Outport  Port=5
  acsExtMdSoftInt : Outport  Port=6  VectorParamsAs1DForOutWhenUnconnected=on
  SwAcsExtRIntCnt : Outport  Port=7
  wires:
  SwLtRclReq/1 -> Subsystem1/1
  SwLtRclReqV/1 -> Subsystem1/2
  SwRtRclReq/1 -> Subsystem4/1
  passCmprtMdHMIReq/1 -> Unit Delay3/1, Relational Operator/1
  Constant2/1 -> Relational Operator/2
  Subsystem4/1 -> ButtonLongPressed/1(modeReq)
  ButtonLongPressed/1(mdReq) -> Logical Operator1/1
  ButtonLongPressed1/1(mdReq) -> Logical Operator1/2
  Subsystem1/1 -> ButtonLongPressed1/1(modeReq)
  ButtonLongPressed1/2(mdInterruptCnt) -> "SwAcsExtLIntCnt "/1, Unit Delay8/1, Equal8/1
  buttonLongPressedThrshhldTm/1 -> [buttonLongPressedThrshhldTm]
  curMode/1 -> [curMode]
  [buttonLongPressedThrshhldTm] -> ButtonLongPressed/2(longPressThrshhldTm)
  [buttonLongPressedThrshhldTm] -> ButtonLongPressed1/2(longPressThrshhldTm)
  Constant5/1 -> ButtonLongPressed2/2(longPressThrshhldTm)
  [curMode] -> ButtonLongPressed2/3(curMdState)
  SRSSlctSwReq/1 -> SRSReq/1
  SRSCnfmSwReq/1 -> ButtonLongPressed2/5(SRSCnfmSwReq), SRSReq/3
  Constant1/1 -> SRSReq/4, ButtonLongPressed2/4(CmpReq)
  SRSActiveValidTm/1 -> SRSReq/2
  SRSReq/1 -> ButtonLongPressed2/1(modeReq)
  ButtonLongPressed2/2(mdInterruptCnt) -> SRSRclIntCnt/1
  SwRtRclReqV/1 -> Subsystem4/2
  ButtonLongPressed/2(mdInterruptCnt) -> SwAcsExtRIntCnt/1, Unit Delay7/1, Equal7/1
  Constant/1 -> Equal1/2, Equal/2
  Unit Delay/1 -> Equal1/1
  Equal/1 -> AND/1
  Equal1/1 -> AND/2
  Logical Operator1/1 -> [SwMdReq]
  [SwMdReq] -> ConfirmRequireSource/1, Logical Operator/1
  AND/1 -> [HMI2LReq]
  Constant3/1 -> Equal3/2, Equal2/2
  Equal2/1 -> AND1/1
  Equal3/1 -> AND1/2
  AND1/1 -> [HMI2RReq]
  [HMI2RReq] -> OR1/2, ConfirmRequireSource/3, Logical Operator/3
  Constant4/1 -> Equal4/2, Equal5/2
  PassAcsMdExtReq/1 -> Unit Delay2/1, Equal4/1
  Equal4/1 -> AND2/1
  Equal5/1 -> AND2/2
  AND2/1 -> [PassAcsMdExtReq]
  Unit Delay1/1 -> Equal3/1
  Unit Delay2/1 -> Equal5/1
  Unit Delay3/1 -> Equal6/1
  Relational Operator/1 -> AND3/1
  Equal6/1 -> AND3/2
  AND3/1 -> [passCmprtMdHMIReq]
  [passCmprtMdHMIReq] -> OR1/4, ConfirmRequireSource/4, Logical Operator/5
  [SRSReq] -> ConfirmRequireSource/6, Logical Operator/6
  [PassAcsMdExtReq] -> ConfirmRequireSource/5, OR1/3, Logical Operator/4
  Logical Operator/1 -> AND4/1, Switch1/1
  AcsMdExtAvl/1 -> Switch2/2, NOT/1, Switch1/2
  Switch1/1 -> Unit Delay4/1, acsExtMdReq/1
  Unit Delay4/1 -> Switch1/3
  NOT/1 -> AND4/2
  AND4/1 -> Notf1ChimeEventStat/1
  Switch2/1 -> Unit Delay5/1, acsExtMdSoftInt/1
  Unit Delay5/1 -> Switch2/3
  OR1/1 -> Switch2/1
  [HMI2LReq] -> ConfirmRequireSource/2, OR1/1, Logical Operator/2
  ConfirmRequireSource/1 -> srcReqTp/1
  SRSMode/1 -> Unit Delay6/1
  Unit Delay6/1 -> ButtonLongPressed2/6(SRSMode)
  ButtonLongPressed2/1(mdReq) -> [SRSReq]
  HMI2LRclReq/1 -> Unit Delay/1, Equal/1
  HMI2RRclReq/1 -> Unit Delay1/1, Equal2/1
  Constant8/1 -> Equal6/2
  Unit Delay7/1 -> Equal7/2
  Unit Delay8/1 -> Equal8/2
  Equal7/1 -> OR/1
  Equal8/1 -> OR/2
  OR/1 -> SWIntSrc/1, Unit Delay9/1, Equal9/1
  Unit Delay9/1 -> Equal9/2
  Equal9/1 -> SWIntSrc/2
  Constant11/1 -> SWIntSrc/3

== system ModeInputHandle/ModelInputHandleRunnable_sys/Subsystem1/Big4SeatMdReq ==
  StPassCmprtMdHMIReqExt2 : Inport
  Big4SeatAvl : Inport  Port=2
  StPassCmprtMdCtrl_Md56_VCUConfig : Inport  Port=3
  AND : Logic  AllPortsSameDT=off  OutDataTypeStr=boolean
  AND10 : Logic  AllPortsSameDT=off  OutDataTypeStr=boolean
  ConfirmRequireSource : MSMLib/ConfirmRequireSource  SystemSampleTime=-1
  Constant : Constant  Value=0  OutDataTypeStr=boolean
  Constant4 : Constant  Value=CmprtMdHMIReqExt2Tp1.CmprtMdHMIReqExt2Tp_Mode56  OutDataTypeStr=Enum:CmprtMdHMIReqExt2Tp1
  Constant9 : Constant  Value=CmprtMdHMIReqExt2Tp1.CmprtMdHMIReqExt2Tp_NoAction  OutDataTypeStr=Enum:CmprtMdHMIReqExt2Tp1
  Equal10 : RelationalOperator  Operator===  OutDataTypeStr=boolean  RndMeth=Simplest
  Ground : Ground
  NOT : Logic  Operator=NOT  AllPortsSameDT=off  OutDataTypeStr=boolean
  Relational Operator3 : RelationalOperator  Operator===  OutDataTypeStr=boolean  RndMeth=Simplest
  Switch : Switch  Criteria=u2 > Threshold
  Switch1 : Switch  Criteria=u2 > Threshold
  Switch2 : Switch  Criteria=u2 > Threshold
  Unit Delay : UnitDelay  SampleTime=-1
  Unit Delay12 : UnitDelay  InitialCondition=j  SampleTime=-1
  Unit Delay6 : UnitDelay  SampleTime=-1
  Big4SeatReq : Outport  VectorParamsAs1DForOutWhenUnconnected=on
  Big4SeatsrcReqTp : Outport  Port=2  VectorParamsAs1DForOutWhenUnconnected=on
  Big4SeatSoftInt : Outport  Port=3
  Big4SeatNotf1ChimeEventStat : Outport  Port=4
  wires:
  Relational Operator3/1 -> AND10/1
  StPassCmprtMdHMIReqExt2/1 -> Unit Delay12/1, Relational Operator3/1
  Constant4/1 -> Relational Operator3/2
  Unit Delay12/1 -> Equal10/1
  Constant9/1 -> Equal10/2
  Equal10/1 -> AND10/2
  Switch1/1 -> Unit Delay/1, Big4SeatReq/1
  ConfirmRequireSource/1 -> Big4SeatsrcReqTp/1
  NOT/1 -> AND/2
  Ground/1 -> ConfirmRequireSource/1, ConfirmRequireSource/5, ConfirmRequireSource/6, ConfirmRequireSource/3, ConfirmRequireSource/2
  [passCmprtMdHMIReq_Big4Seat] -> Switch2/1, ConfirmRequireSource/4, Switch1/1, AND/1
  AND/1 -> Big4SeatNotf1ChimeEventStat/1
  Unit Delay6/1 -> Switch2/3
  Switch2/1 -> Big4SeatSoftInt/1, Unit Delay6/1
  Unit Delay/1 -> Switch1/3
  Big4SeatAvl/1 -> Switch2/2, NOT/1, Switch1/2
  StPassCmprtMdCtrl_Md56_VCUConfig/1 -> Switch/2
  AND10/1 -> Switch/1
  Switch/1 -> [passCmprtMdHMIReq_Big4Seat]
  Constant/1 -> Switch/3

== system ModeInputHandle/ModelInputHandleRunnable_sys/Subsystem1/ExVIPMdReq  ==
  StPassCmprtMdHMIReqExt2 : Inport
  ExVipRMdAvl : Inport  Port=2
  ExVipROutMdAvl : Inport  Port=3
  StPassCmprtMdCtrl_Md57_VCUConfig : Inport  Port=4
  StPassCmprtMdCtrl_Md58_VCUConfig : Inport  Port=5
  AND{,1..2,10} (4 alike) : Logic  AllPortsSameDT=off  OutDataTypeStr=boolean
  ConfirmRequireSource : MSMLib/ConfirmRequireSource  SystemSampleTime=-1
  ConfirmRequireSource1 : MSMLib/ConfirmRequireSource  SystemSampleTime=-1
  Constant : Constant  Value=0  OutDataTypeStr=boolean
  Constant1 : Constant  Value=CmprtMdHMIReqExt2Tp1.CmprtMdHMIReqExt2Tp_Mode58  OutDataTypeStr=Enum:CmprtMdHMIReqExt2Tp1
  Constant2 : Constant  Value=CmprtMdHMIReqExt2Tp1.CmprtMdHMIReqExt2Tp_NoAction  OutDataTypeStr=Enum:CmprtMdHMIReqExt2Tp1
  Constant3 : Constant  Value=0  OutDataTypeStr=boolean
  Constant4 : Constant  Value=CmprtMdHMIReqExt2Tp1.CmprtMdHMIReqExt2Tp_Mode57  OutDataTypeStr=Enum:CmprtMdHMIReqExt2Tp1
  Constant9 : Constant  Value=CmprtMdHMIReqExt2Tp1.CmprtMdHMIReqExt2Tp_NoAction  OutDataTypeStr=Enum:CmprtMdHMIReqExt2Tp1
  Equal1 : RelationalOperator  Operator===  OutDataTypeStr=boolean  RndMeth=Simplest
  Equal10 : RelationalOperator  Operator===  OutDataTypeStr=boolean  RndMeth=Simplest
  Ground : Ground
  Ground1 : Ground
  NOT : Logic  Operator=NOT  AllPortsSameDT=off  OutDataTypeStr=boolean
  NOT1 : Logic  Operator=NOT  AllPortsSameDT=off  OutDataTypeStr=boolean
  Relational Operator1 : RelationalOperator  Operator===  OutDataTypeStr=boolean  RndMeth=Simplest
  Relational Operator3 : RelationalOperator  Operator===  OutDataTypeStr=boolean  RndMeth=Simplest
  Switch{,1..5} (6 alike) : Switch  Criteria=u2 > Threshold
  Unit Delay{,2..3,6} (4 alike) : UnitDelay  SampleTime=-1
  Unit Delay1 : UnitDelay  InitialCondition=j  SampleTime=-1
  Unit Delay12 : UnitDelay  InitialCondition=j  SampleTime=-1
  ExVIPRReq : Outport  VectorParamsAs1DForOutWhenUnconnected=on
  ExVIPRsrcReqTp : Outport  Port=2  VectorParamsAs1DForOutWhenUnconnected=on
  ExVIPRSoftInt : Outport  Port=3
  ExVIPRNotf1ChimeEventStat : Outport  Port=4
  ExVIPROutReq : Outport  Port=5  VectorParamsAs1DForOutWhenUnconnected=on
  ExVIPROutsrcReqTp : Outport  Port=6  VectorParamsAs1DForOutWhenUnconnected=on
  ExVIPROutSoftInt : Outport  Port=7
  ExVIPROutNotf1ChimeEventStat : Outport  Port=8
  wires:
  Unit Delay12/1 -> Equal10/1
  Constant4/1 -> Relational Operator3/2
  Constant9/1 -> Equal10/2
  Equal10/1 -> AND10/2
  Relational Operator3/1 -> AND10/1
  Switch1/1 -> Unit Delay/1, ExVIPRReq/1
  Unit Delay/1 -> Switch1/3
  NOT/1 -> AND/2
  Unit Delay6/1 -> Switch2/3
  Switch2/1 -> ExVIPRSoftInt/1, Unit Delay6/1
  [passCmprtMdHMIReq_ExVIPR] -> Switch2/1, ConfirmRequireSource/4, Switch1/1, AND/1
  AND/1 -> ExVIPRNotf1ChimeEventStat/1
  ConfirmRequireSource/1 -> ExVIPRsrcReqTp/1
  Ground/1 -> ConfirmRequireSource/1, ConfirmRequireSource/5, ConfirmRequireSource/6, ConfirmRequireSource/3, ConfirmRequireSource/2
  ExVipRMdAvl/1 -> Switch2/2, NOT/1, Switch1/2
  [StPassCmprtMdHMIReqExt2] -> Unit Delay1/1, Relational Operator1/1
  Constant1/1 -> Relational Operator1/2
  Constant2/1 -> Equal1/2
  Equal1/1 -> AND1/2
  Unit Delay1/1 -> Equal1/1
  Relational Operator1/1 -> AND1/1
  StPassCmprtMdHMIReqExt2/1 -> [StPassCmprtMdHMIReqExt2]
  [StPassCmprtMdHMIReqExt2] -> Unit Delay12/1, Relational Operator3/1
  ConfirmRequireSource1/1 -> ExVIPROutsrcReqTp/1
  [passCmprtMdHMIReq_ExVIPROut] -> Switch4/1, ConfirmRequireSource1/4, Switch3/1, AND2/1
  Ground1/1 -> ConfirmRequireSource1/1, ConfirmRequireSource1/5, ConfirmRequireSource1/6, ConfirmRequireSource1/3, ConfirmRequireSource1/2
  AND2/1 -> ExVIPROutNotf1ChimeEventStat/1
  Unit Delay2/1 -> Switch3/3
  NOT1/1 -> AND2/2
  Unit Delay3/1 -> Switch4/3
  Switch4/1 -> ExVIPROutSoftInt/1, Unit Delay3/1
  Switch3/1 -> Unit Delay2/1, ExVIPROutReq/1
  ExVipROutMdAvl/1 -> Switch4/2, NOT1/1, Switch3/2
  StPassCmprtMdCtrl_Md57_VCUConfig/1 -> Switch/2
  AND10/1 -> Switch/1
  Switch/1 -> [passCmprtMdHMIReq_ExVIPR]
  Constant/1 -> Switch/3
  AND1/1 -> Switch5/1
  StPassCmprtMdCtrl_Md58_VCUConfig/1 -> Switch5/2
  Constant3/1 -> Switch5/3
  Switch5/1 -> [passCmprtMdHMIReq_ExVIPROut]
